simulink model "test_trigger"  (R2018a)
settings: Solver=VariableStepAuto  StartTime=0.0  StopTime=0.001  RelTol=1e-3
values from neighbouring files (symbols this model uses):
  safty_height = (ptCloud.ZLimits(2) - ptCloud.ZLimits(1)) * 1000    [final_test.m]    (also in main_file.m)
  transfer_array = zeros(1,30)    [final_test.m]    (also in main_file.m = calc_corr_arr(transfer_array, v_m))
  v_m = 0.5*median(vel_norm(end-4:end)) + 0.5*mean(vel_norm(end-4:end))    [final_test.m]    (also in main_file.m = mean(vel_norm(end-3:end)) * 1000; vel_measurement_final.m = mean(vel_norm(end-3:end)); vel_test_25_3_2019.m = mean(vel_norm(end-3:end)))
libraries: TcAdsLib x4
settings Model: Creator=bschumann  LastModifiedBy=bschumann

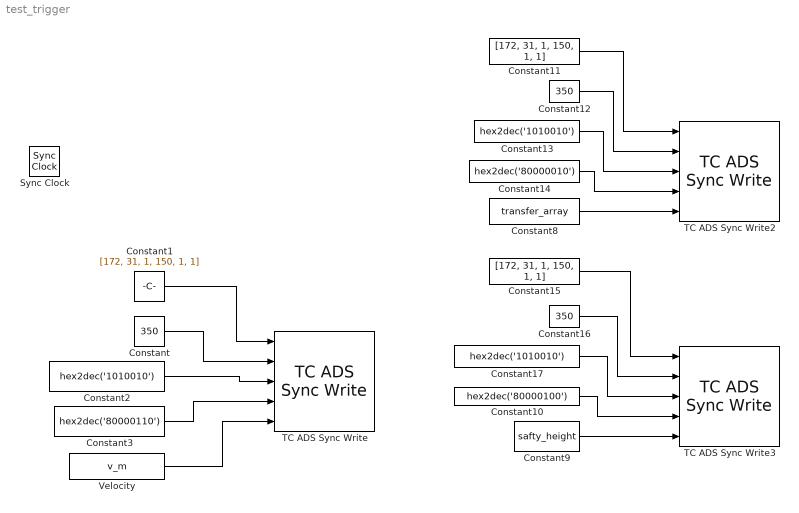
== system test_trigger ==
  Constant : Constant  Value=350  OutDataTypeStr=uint16
  Constant1 : Constant  Value=[172, 31, 1, 150, 1, 1]  OutDataTypeStr=uint8
  Constant10 : Constant  Value=hex2dec('80000100')  OutDataTypeStr=uint32
  Constant11 : Constant  Value=[172, 31, 1, 150, 1, 1]  OutDataTypeStr=uint8
  Constant12 : Constant  Value=350  OutDataTypeStr=uint16
  Constant13 : Constant  Value=hex2dec('1010010')  OutDataTypeStr=uint32
  Constant14 : Constant  Value=hex2dec('80000010')  OutDataTypeStr=uint32
  Constant15 : Constant  Value=[172, 31, 1, 150, 1, 1]  OutDataTypeStr=uint8
  Constant16 : Constant  Value=350  OutDataTypeStr=uint16
  Constant17 : Constant  Value=hex2dec('1010010')  OutDataTypeStr=uint32
  Constant2 : Constant  Value=hex2dec('1010010')  OutDataTypeStr=uint32
  Constant3 : Constant  Value=hex2dec('80000110')  OutDataTypeStr=uint32
  Constant8 : Constant  Value=transfer_array
  Constant9 : Constant  Value=safty_height
  Sync Clock : TcAdsLib/Utilities/Sync Clock  OutputPortSelect=None  InputPortSelect=None
      settings: SourceProductName=Beckhoff TwinCAT ADS Interface
  TC ADS Sync Write : TcAdsLib/Synchronous/TC ADS Sync Write  SampleTime=-1  AbortSimulationOnAdsError=off  WriteDataType=double  WriteDataDim=1  WriteDataColToRowMajor=on  AdsTimeout=1  DirectFeedThrough=off  CreateSignalLabels=on  CodeGenConnectType=DataArea (OutputSrc)
      settings: SourceProductName=Beckhoff TwinCAT ADS Interface
  TC ADS Sync Write2 : TcAdsLib/Synchronous/TC ADS Sync Write  SampleTime=-1  AbortSimulationOnAdsError=off  WriteDataType=double  WriteDataDim=30  WriteDataColToRowMajor=on  AdsTimeout=1  DirectFeedThrough=off  CreateSignalLabels=on  CodeGenConnectType=DataArea (OutputSrc)
      settings: SourceProductName=Beckhoff TwinCAT ADS Interface
  TC ADS Sync Write3 : TcAdsLib/Synchronous/TC ADS Sync Write  SampleTime=-1  AbortSimulationOnAdsError=off  WriteDataType=double  WriteDataDim=1  WriteDataColToRowMajor=on  AdsTimeout=1  DirectFeedThrough=off  CreateSignalLabels=on  CodeGenConnectType=DataArea (OutputSrc)
      settings: SourceProductName=Beckhoff TwinCAT ADS Interface
  Velocity : Constant  Value=v_m
  wires:
  Constant3/1 -> TC ADS Sync Write/4
  Constant1/1 -> TC ADS Sync Write/1
  Velocity/1 -> TC ADS Sync Write/5
  Constant2/1 -> TC ADS Sync Write/3
  Constant/1 -> TC ADS Sync Write/2
  Constant9/1 -> TC ADS Sync Write3/5
  Constant14/1 -> TC ADS Sync Write2/4
  Constant16/1 -> TC ADS Sync Write3/2
  Constant8/1 -> TC ADS Sync Write2/5
  Constant13/1 -> TC ADS Sync Write2/3
  Constant15/1 -> TC ADS Sync Write3/1
  Constant12/1 -> TC ADS Sync Write2/2
  Constant17/1 -> TC ADS Sync Write3/3
  Constant10/1 -> TC ADS Sync Write3/4
  Constant11/1 -> TC ADS Sync Write2/1
